simulink model "KillerWhaleModel"  (R2020b)
settings: Solver=ode15s  StartTime=0.0  StopTime=10.0  MaxStep=0.01  RelTol=1e-3
model workspace: external: MATLAB File KillerWhaleParams.m (data not in the file)
undefined symbols (not defined in the file or in its folder): frontParams, rearParams, standParams, X, Y, Z
libraries: sm_lib x4076, nesl_utility x6
(part 4 of 62)

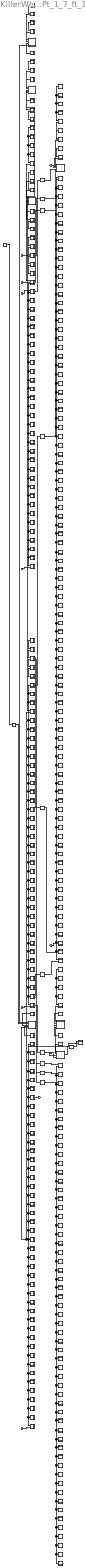
== system KillerWhaleModel/RearLinkage/Tail_Linkage_Pt_1_7_ft_1 ==
  Bracket_10_RIGID : Subsystem
  Bracket_11_RIGID : Subsystem
  Bracket_12_RIGID : Subsystem
  Bracket_13_RIGID : Subsystem
  Bracket_14_RIGID : Subsystem
  Bracket_15_RIGID : Subsystem
  Bracket_16_RIGID : Subsystem
  Bracket_17_RIGID : Subsystem
  Bracket_18_RIGID : Subsystem
  Bracket_19_RIGID : Subsystem
  Bracket_1_RIGID : Subsystem
  Bracket_1_RIGID1 : Subsystem
  Bracket_20_RIGID : Subsystem
  Bracket_21_RIGID : Subsystem
  Bracket_22_RIGID : Subsystem
  Bracket_2_RIGID : Subsystem
  Bracket_2_RIGID1 : Subsystem
  Bracket_3_RIGID : Subsystem
  Bracket_4_RIGID : Subsystem
  Bracket_5_RIGID : Subsystem
  Bracket_6_RIGID : Subsystem
  Bracket_7_RIGID : Subsystem
  Bracket_8_RIGID : Subsystem
  Bracket_9_RIGID : Subsystem
  Cylindrical3 : sm_lib/Joints/Cylindrical Joint  JointMode=Normal  SenseConstraintForce=off  SenseConstraintForceX=off  SenseConstraintForceY=off  SenseConstraintForceZ=off  SenseConstraintTorque=off  SenseConstraintTorqueX=off  SenseConstraintTorqueY=off  SenseConstraintTorqueZ=off  SenseTotalForce=off  SenseTotalForceX=off  SenseTotalForceY=off  SenseTotalForceZ=off  SenseTotalTorque=off  SenseTotalTorqueX=off  SenseTotalTorqueY=off  SenseTotalTorqueZ=off  CompositeWrenchDir=FollowerOnBase  CompositeWrenchFrame=BaseFrame  PzEquilibriumPosition=0  PzEquilibriumPositionUnits=m  PzSpringStiffness=0  PzSpringStiffnessUnits=N/m  PzDampingCoefficient=0  PzDampingCoefficientUnits=N/(m/s)  PzTorqueActuationMode=NoTorque  PzMotionActuationMode=ComputedMotion  PzSensePosition=off  PzSenseVelocity=off  PzSenseAcceleration=off  PzSenseTorqueForce=off  PzSenseLowerLimitTorqueForce=off  PzSenseUpperLimitTorqueForce=off  PzLowerLimitSpecify=off  PzLowerLimitBound=-1  PzLowerLimitBoundUnits=m  PzLowerLimitStiffness=1e6  PzLowerLimitStiffnessUnits=N/m  PzLowerLimitDamping=1e3  PzLowerLimitDampingUnits=N/(m/s)  PzLowerLimitTransitionRegionWidth=1e-4  PzLowerLimitTransitionRegionWidthUnits=m  PzUpperLimitSpecify=off  PzUpperLimitBound=1  PzUpperLimitBoundUnits=m  PzUpperLimitStiffness=1e6  PzUpperLimitStiffnessUnits=N/m  PzUpperLimitDamping=1e3  PzUpperLimitDampingUnits=N/(m/s)  PzUpperLimitTransitionRegionWidth=1e-4  PzUpperLimitTransitionRegionWidthUnits=m  PzPositionTargetSpecify=off  PzPositionTargetPriority=High  PzPositionTargetValue=0  PzPositionTargetValueUnits=m  PzVelocityTargetSpecify=off  PzVelocityTargetPriority=High  PzVelocityTargetValue=0  PzVelocityTargetValueUnits=m/s  RzEquilibriumPosition=0  RzEquilibriumPositionUnits=deg  RzSpringStiffness=0  RzSpringStiffnessUnits=N*m/deg  RzDampingCoefficient=0  RzDampingCoefficientUnits=N*m/(deg/s)  RzTorqueActuationMode=NoTorque  RzMotionActuationMode=ComputedMotion  RzSensePosition=off  RzSenseVelocity=off  RzSenseAcceleration=off  RzSenseTorqueForce=off  RzSenseLowerLimitTorqueForce=off  RzSenseUpperLimitTorqueForce=off  RzLowerLimitSpecify=off  RzLowerLimitBound=-90  RzLowerLimitBoundUnits=deg  RzLowerLimitStiffness=1e4  RzLowerLimitStiffnessUnits=N*m/deg  RzLowerLimitDamping=10  RzLowerLimitDampingUnits=N*m/(deg/s)  RzLowerLimitTransitionRegionWidth=0.1  RzLowerLimitTransitionRegionWidthUnits=deg  RzUpperLimitSpecify=off  RzUpperLimitBound=90  RzUpperLimitBoundUnits=deg  RzUpperLimitStiffness=1e4  RzUpperLimitStiffnessUnits=N*m/deg  RzUpperLimitDamping=10  RzUpperLimitDampingUnits=N*m/(deg/s)  RzUpperLimitTransitionRegionWidth=0.1  RzUpperLimitTransitionRegionWidthUnits=deg  RzPositionTargetSpecify=off  RzPositionTargetPriority=High  RzPositionTargetValue=0  RzPositionTargetValueUnits=deg  RzVelocityTargetSpecify=off  RzVelocityTargetPriority=High  RzVelocityTargetValue=0  RzVelocityTargetValueUnits=deg/s
  Cylindrical4 : sm_lib/Joints/Cylindrical Joint  JointMode=Normal  SenseConstraintForce=off  SenseConstraintForceX=off  SenseConstraintForceY=off  SenseConstraintForceZ=off  SenseConstraintTorque=off  SenseConstraintTorqueX=off  SenseConstraintTorqueY=off  SenseConstraintTorqueZ=off  SenseTotalForce=off  SenseTotalForceX=off  SenseTotalForceY=off  SenseTotalForceZ=off  SenseTotalTorque=off  SenseTotalTorqueX=off  SenseTotalTorqueY=off  SenseTotalTorqueZ=off  CompositeWrenchDir=FollowerOnBase  CompositeWrenchFrame=BaseFrame  PzEquilibriumPosition=0  PzEquilibriumPositionUnits=m  PzSpringStiffness=0  PzSpringStiffnessUnits=N/m  PzDampingCoefficient=0  PzDampingCoefficientUnits=N/(m/s)  PzTorqueActuationMode=NoTorque  PzMotionActuationMode=ComputedMotion  PzSensePosition=off  PzSenseVelocity=off  PzSenseAcceleration=off  PzSenseTorqueForce=off  PzSenseLowerLimitTorqueForce=off  PzSenseUpperLimitTorqueForce=off  PzLowerLimitSpecify=off  PzLowerLimitBound=-1  PzLowerLimitBoundUnits=m  PzLowerLimitStiffness=1e6  PzLowerLimitStiffnessUnits=N/m  PzLowerLimitDamping=1e3  PzLowerLimitDampingUnits=N/(m/s)  PzLowerLimitTransitionRegionWidth=1e-4  PzLowerLimitTransitionRegionWidthUnits=m  PzUpperLimitSpecify=off  PzUpperLimitBound=1  PzUpperLimitBoundUnits=m  PzUpperLimitStiffness=1e6  PzUpperLimitStiffnessUnits=N/m  PzUpperLimitDamping=1e3  PzUpperLimitDampingUnits=N/(m/s)  PzUpperLimitTransitionRegionWidth=1e-4  PzUpperLimitTransitionRegionWidthUnits=m  PzPositionTargetSpecify=off  PzPositionTargetPriority=High  PzPositionTargetValue=0  PzPositionTargetValueUnits=m  PzVelocityTargetSpecify=off  PzVelocityTargetPriority=High  PzVelocityTargetValue=0  PzVelocityTargetValueUnits=m/s  RzEquilibriumPosition=0  RzEquilibriumPositionUnits=deg  RzSpringStiffness=0  RzSpringStiffnessUnits=N*m/deg  RzDampingCoefficient=0  RzDampingCoefficientUnits=N*m/(deg/s)  RzTorqueActuationMode=NoTorque  RzMotionActuationMode=ComputedMotion  RzSensePosition=off  RzSenseVelocity=off  RzSenseAcceleration=off  RzSenseTorqueForce=off  RzSenseLowerLimitTorqueForce=off  RzSenseUpperLimitTorqueForce=off  RzLowerLimitSpecify=off  RzLowerLimitBound=-90  RzLowerLimitBoundUnits=deg  RzLowerLimitStiffness=1e4  RzLowerLimitStiffnessUnits=N*m/deg  RzLowerLimitDamping=10  RzLowerLimitDampingUnits=N*m/(deg/s)  RzLowerLimitTransitionRegionWidth=0.1  RzLowerLimitTransitionRegionWidthUnits=deg  RzUpperLimitSpecify=off  RzUpperLimitBound=90  RzUpperLimitBoundUnits=deg  RzUpperLimitStiffness=1e4  RzUpperLimitStiffnessUnits=N*m/deg  RzUpperLimitDamping=10  RzUpperLimitDampingUnits=N*m/(deg/s)  RzUpperLimitTransitionRegionWidth=0.1  RzUpperLimitTransitionRegionWidthUnits=deg  RzPositionTargetSpecify=off  RzPositionTargetPriority=High  RzPositionTargetValue=0  RzPositionTargetValueUnits=deg  RzVelocityTargetSpecify=off  RzVelocityTargetPriority=High  RzVelocityTargetValue=0  RzVelocityTargetValueUnits=deg/s
  Cylindrical5 : sm_lib/Joints/Cylindrical Joint  JointMode=Normal  SenseConstraintForce=off  SenseConstraintForceX=off  SenseConstraintForceY=off  SenseConstraintForceZ=off  SenseConstraintTorque=off  SenseConstraintTorqueX=off  SenseConstraintTorqueY=off  SenseConstraintTorqueZ=off  SenseTotalForce=off  SenseTotalForceX=off  SenseTotalForceY=off  SenseTotalForceZ=off  SenseTotalTorque=off  SenseTotalTorqueX=off  SenseTotalTorqueY=off  SenseTotalTorqueZ=off  CompositeWrenchDir=FollowerOnBase  CompositeWrenchFrame=BaseFrame  PzEquilibriumPosition=0  PzEquilibriumPositionUnits=m  PzSpringStiffness=0  PzSpringStiffnessUnits=N/m  PzDampingCoefficient=0  PzDampingCoefficientUnits=N/(m/s)  PzTorqueActuationMode=NoTorque  PzMotionActuationMode=ComputedMotion  PzSensePosition=off  PzSenseVelocity=off  PzSenseAcceleration=off  PzSenseTorqueForce=off  PzSenseLowerLimitTorqueForce=off  PzSenseUpperLimitTorqueForce=off  PzLowerLimitSpecify=off  PzLowerLimitBound=-1  PzLowerLimitBoundUnits=m  PzLowerLimitStiffness=1e6  PzLowerLimitStiffnessUnits=N/m  PzLowerLimitDamping=1e3  PzLowerLimitDampingUnits=N/(m/s)  PzLowerLimitTransitionRegionWidth=1e-4  PzLowerLimitTransitionRegionWidthUnits=m  PzUpperLimitSpecify=off  PzUpperLimitBound=1  PzUpperLimitBoundUnits=m  PzUpperLimitStiffness=1e6  PzUpperLimitStiffnessUnits=N/m  PzUpperLimitDamping=1e3  PzUpperLimitDampingUnits=N/(m/s)  PzUpperLimitTransitionRegionWidth=1e-4  PzUpperLimitTransitionRegionWidthUnits=m  PzPositionTargetSpecify=off  PzPositionTargetPriority=High  PzPositionTargetValue=0  PzPositionTargetValueUnits=m  PzVelocityTargetSpecify=off  PzVelocityTargetPriority=High  PzVelocityTargetValue=0  PzVelocityTargetValueUnits=m/s  RzEquilibriumPosition=0  RzEquilibriumPositionUnits=deg  RzSpringStiffness=0  RzSpringStiffnessUnits=N*m/deg  RzDampingCoefficient=0  RzDampingCoefficientUnits=N*m/(deg/s)  RzTorqueActuationMode=NoTorque  RzMotionActuationMode=ComputedMotion  RzSensePosition=off  RzSenseVelocity=off  RzSenseAcceleration=off  RzSenseTorqueForce=off  RzSenseLowerLimitTorqueForce=off  RzSenseUpperLimitTorqueForce=off  RzLowerLimitSpecify=off  RzLowerLimitBound=-90  RzLowerLimitBoundUnits=deg  RzLowerLimitStiffness=1e4  RzLowerLimitStiffnessUnits=N*m/deg  RzLowerLimitDamping=10  RzLowerLimitDampingUnits=N*m/(deg/s)  RzLowerLimitTransitionRegionWidth=0.1  RzLowerLimitTransitionRegionWidthUnits=deg  RzUpperLimitSpecify=off  RzUpperLimitBound=90  RzUpperLimitBoundUnits=deg  RzUpperLimitStiffness=1e4  RzUpperLimitStiffnessUnits=N*m/deg  RzUpperLimitDamping=10  RzUpperLimitDampingUnits=N*m/(deg/s)  RzUpperLimitTransitionRegionWidth=0.1  RzUpperLimitTransitionRegionWidthUnits=deg  RzPositionTargetSpecify=off  RzPositionTargetPriority=High  RzPositionTargetValue=0  RzPositionTargetValueUnits=deg  RzVelocityTargetSpecify=off  RzVelocityTargetPriority=High  RzVelocityTargetValue=0  RzVelocityTargetValueUnits=deg/s
  Frame_Part_1_RIGID : Subsystem
  Frame_Part_1_RIGID1 : Subsystem
  Frame_Part_1_RIGID2 : Subsystem
  Frame_Part_2_RIGID : Subsystem
  Frame_Part_2_RIGID1 : Subsystem
  Frame_Part_2_RIGID2 : Subsystem
  Hinge_10_RIGID : Subsystem
  Hinge_11_RIGID : Subsystem
  Hinge_13_RIGID : Subsystem
  Hinge_1_RIGID : Subsystem
  Hinge_1_RIGID1 : Subsystem
  Hinge_1_RIGID2 : Subsystem
  Hinge_2_RIGID : Subsystem
  Hinge_3_RIGID : Subsystem
  Hinge_4_RIGID : Subsystem
  Hinge_5_RIGID : Subsystem
  Hinge_6_RIGID : Subsystem
  Hinge_7_RIGID : Subsystem
  Hinge_8_RIGID : Subsystem
  Hinge_9_RIGID : Subsystem
  Lock_tabs_1_RIGID : Subsystem
  Lock_tabs_1_RIGID1 : Subsystem
  Lock_tabs_1_RIGID10 : Subsystem
  Lock_tabs_1_RIGID11 : Subsystem
  Lock_tabs_1_RIGID12 : Subsystem
  Lock_tabs_1_RIGID13 : Subsystem
  Lock_tabs_1_RIGID2 : Subsystem
  Lock_tabs_1_RIGID3 : Subsystem
  Lock_tabs_1_RIGID4 : Subsystem
  Lock_tabs_1_RIGID5 : Subsystem
  Lock_tabs_1_RIGID6 : Subsystem
  Lock_tabs_1_RIGID7 : Subsystem
  Lock_tabs_1_RIGID8 : Subsystem
  Lock_tabs_1_RIGID9 : Subsystem
  ReferenceFrame : sm_lib/Frames and Transforms/Reference Frame
  Revolute1 : sm_lib/Joints/Revolute Joint  JointMode=Normal  SenseConstraintForce=off  SenseConstraintForceX=off  SenseConstraintForceY=off  SenseConstraintForceZ=off  SenseConstraintTorque=off  SenseConstraintTorqueX=off  SenseConstraintTorqueY=off  SenseConstraintTorqueZ=off  SenseTotalForce=off  SenseTotalForceX=off  SenseTotalForceY=off  SenseTotalForceZ=off  SenseTotalTorque=off  SenseTotalTorqueX=off  SenseTotalTorqueY=off  SenseTotalTorqueZ=off  CompositeWrenchDir=FollowerOnBase  CompositeWrenchFrame=BaseFrame  EquilibriumPosition=0  EquilibriumPositionUnits=deg  SpringStiffness=0  SpringStiffnessUnits=N*m/deg  DampingCoefficient=0  DampingCoefficientUnits=N*m/(deg/s)  TorqueActuationMode=NoTorque  MotionActuationMode=ComputedMotion  SensePosition=off  SenseVelocity=off  SenseAcceleration=off  SenseTorqueForce=off  SenseLowerLimitTorqueForce=off  SenseUpperLimitTorqueForce=off  LowerLimitSpecify=off  LowerLimitBound=-90  LowerLimitBoundUnits=deg  LowerLimitStiffness=1e4  LowerLimitStiffnessUnits=N*m/deg  LowerLimitDamping=10  LowerLimitDampingUnits=N*m/(deg/s)  LowerLimitTransitionRegionWidth=0.1  LowerLimitTransitionRegionWidthUnits=deg  UpperLimitSpecify=off  UpperLimitBound=90  UpperLimitBoundUnits=deg  UpperLimitStiffness=1e4  UpperLimitStiffnessUnits=N*m/deg  UpperLimitDamping=10  UpperLimitDampingUnits=N*m/(deg/s)  UpperLimitTransitionRegionWidth=0.1  UpperLimitTransitionRegionWidthUnits=deg  PositionTargetSpecify=on  PositionTargetPriority=Low  PositionTargetValue=rearParams.RevoluteJoint(18).Rz.Pos  PositionTargetValueUnits=deg  VelocityTargetSpecify=off  VelocityTargetPriority=High  VelocityTargetValue=0  VelocityTargetValueUnits=deg/s
  Revolute11 : sm_lib/Joints/Revolute Joint  JointMode=Normal  SenseConstraintForce=off  SenseConstraintForceX=off  SenseConstraintForceY=off  SenseConstraintForceZ=off  SenseConstraintTorque=off  SenseConstraintTorqueX=off  SenseConstraintTorqueY=off  SenseConstraintTorqueZ=off  SenseTotalForce=off  SenseTotalForceX=off  SenseTotalForceY=off  SenseTotalForceZ=off  SenseTotalTorque=off  SenseTotalTorqueX=off  SenseTotalTorqueY=off  SenseTotalTorqueZ=off  CompositeWrenchDir=FollowerOnBase  CompositeWrenchFrame=BaseFrame  EquilibriumPosition=0  EquilibriumPositionUnits=deg  SpringStiffness=0  SpringStiffnessUnits=N*m/deg  DampingCoefficient=0  DampingCoefficientUnits=N*m/(deg/s)  TorqueActuationMode=NoTorque  MotionActuationMode=ComputedMotion  SensePosition=off  SenseVelocity=off  SenseAcceleration=off  SenseTorqueForce=off  SenseLowerLimitTorqueForce=off  SenseUpperLimitTorqueForce=off  LowerLimitSpecify=off  LowerLimitBound=-90  LowerLimitBoundUnits=deg  LowerLimitStiffness=1e4  LowerLimitStiffnessUnits=N*m/deg  LowerLimitDamping=10  LowerLimitDampingUnits=N*m/(deg/s)  LowerLimitTransitionRegionWidth=0.1  LowerLimitTransitionRegionWidthUnits=deg  UpperLimitSpecify=off  UpperLimitBound=90  UpperLimitBoundUnits=deg  UpperLimitStiffness=1e4  UpperLimitStiffnessUnits=N*m/deg  UpperLimitDamping=10  UpperLimitDampingUnits=N*m/(deg/s)  UpperLimitTransitionRegionWidth=0.1  UpperLimitTransitionRegionWidthUnits=deg  PositionTargetSpecify=on  PositionTargetPriority=Low  PositionTargetValue=rearParams.RevoluteJoint(16).Rz.Pos  PositionTargetValueUnits=deg  VelocityTargetSpecify=off  VelocityTargetPriority=High  VelocityTargetValue=0  VelocityTargetValueUnits=deg/s
  Revolute2 : sm_lib/Joints/Revolute Joint  JointMode=Normal  SenseConstraintForce=off  SenseConstraintForceX=off  SenseConstraintForceY=off  SenseConstraintForceZ=off  SenseConstraintTorque=off  SenseConstraintTorqueX=off  SenseConstraintTorqueY=off  SenseConstraintTorqueZ=off  SenseTotalForce=off  SenseTotalForceX=off  SenseTotalForceY=off  SenseTotalForceZ=off  SenseTotalTorque=off  SenseTotalTorqueX=off  SenseTotalTorqueY=off  SenseTotalTorqueZ=off  CompositeWrenchDir=FollowerOnBase  CompositeWrenchFrame=BaseFrame  EquilibriumPosition=0  EquilibriumPositionUnits=deg  SpringStiffness=0  SpringStiffnessUnits=N*m/deg  DampingCoefficient=0  DampingCoefficientUnits=N*m/(deg/s)  TorqueActuationMode=NoTorque  MotionActuationMode=ComputedMotion  SensePosition=off  SenseVelocity=off  SenseAcceleration=off  SenseTorqueForce=off  SenseLowerLimitTorqueForce=off  SenseUpperLimitTorqueForce=off  LowerLimitSpecify=off  LowerLimitBound=-90  LowerLimitBoundUnits=deg  LowerLimitStiffness=1e4  LowerLimitStiffnessUnits=N*m/deg  LowerLimitDamping=10  LowerLimitDampingUnits=N*m/(deg/s)  LowerLimitTransitionRegionWidth=0.1  LowerLimitTransitionRegionWidthUnits=deg  UpperLimitSpecify=off  UpperLimitBound=90  UpperLimitBoundUnits=deg  UpperLimitStiffness=1e4  UpperLimitStiffnessUnits=N*m/deg  UpperLimitDamping=10  UpperLimitDampingUnits=N*m/(deg/s)  UpperLimitTransitionRegionWidth=0.1  UpperLimitTransitionRegionWidthUnits=deg  PositionTargetSpecify=off  PositionTargetPriority=High  PositionTargetValue=0  PositionTargetValueUnits=deg  VelocityTargetSpecify=off  VelocityTargetPriority=High  VelocityTargetValue=0  VelocityTargetValueUnits=deg/s
  Revolute3 : sm_lib/Joints/Revolute Joint  JointMode=Normal  SenseConstraintForce=off  SenseConstraintForceX=off  SenseConstraintForceY=off  SenseConstraintForceZ=off  SenseConstraintTorque=off  SenseConstraintTorqueX=off  SenseConstraintTorqueY=off  SenseConstraintTorqueZ=off  SenseTotalForce=off  SenseTotalForceX=off  SenseTotalForceY=off  SenseTotalForceZ=off  SenseTotalTorque=off  SenseTotalTorqueX=off  SenseTotalTorqueY=off  SenseTotalTorqueZ=off  CompositeWrenchDir=FollowerOnBase  CompositeWrenchFrame=BaseFrame  EquilibriumPosition=0  EquilibriumPositionUnits=deg  SpringStiffness=0  SpringStiffnessUnits=N*m/deg  DampingCoefficient=0  DampingCoefficientUnits=N*m/(deg/s)  TorqueActuationMode=NoTorque  MotionActuationMode=ComputedMotion  SensePosition=off  SenseVelocity=off  SenseAcceleration=off  SenseTorqueForce=off  SenseLowerLimitTorqueForce=off  SenseUpperLimitTorqueForce=off  LowerLimitSpecify=off  LowerLimitBound=-90  LowerLimitBoundUnits=deg  LowerLimitStiffness=1e4  LowerLimitStiffnessUnits=N*m/deg  LowerLimitDamping=10  LowerLimitDampingUnits=N*m/(deg/s)  LowerLimitTransitionRegionWidth=0.1  LowerLimitTransitionRegionWidthUnits=deg  UpperLimitSpecify=off  UpperLimitBound=90  UpperLimitBoundUnits=deg  UpperLimitStiffness=1e4  UpperLimitStiffnessUnits=N*m/deg  UpperLimitDamping=10  UpperLimitDampingUnits=N*m/(deg/s)  UpperLimitTransitionRegionWidth=0.1  UpperLimitTransitionRegionWidthUnits=deg  PositionTargetSpecify=on  PositionTargetPriority=Low  PositionTargetValue=rearParams.RevoluteJoint(15).Rz.Pos  PositionTargetValueUnits=deg  VelocityTargetSpecify=off  VelocityTargetPriority=High  VelocityTargetValue=0  VelocityTargetValueUnits=deg/s
  Revolute4 : sm_lib/Joints/Revolute Joint  JointMode=Normal  SenseConstraintForce=off  SenseConstraintForceX=off  SenseConstraintForceY=off  SenseConstraintForceZ=off  SenseConstraintTorque=off  SenseConstraintTorqueX=off  SenseConstraintTorqueY=off  SenseConstraintTorqueZ=off  SenseTotalForce=off  SenseTotalForceX=off  SenseTotalForceY=off  SenseTotalForceZ=off  SenseTotalTorque=off  SenseTotalTorqueX=off  SenseTotalTorqueY=off  SenseTotalTorqueZ=off  CompositeWrenchDir=FollowerOnBase  CompositeWrenchFrame=BaseFrame  EquilibriumPosition=0  EquilibriumPositionUnits=deg  SpringStiffness=0  SpringStiffnessUnits=N*m/deg  DampingCoefficient=0  DampingCoefficientUnits=N*m/(deg/s)  TorqueActuationMode=NoTorque  MotionActuationMode=ComputedMotion  SensePosition=off  SenseVelocity=off  SenseAcceleration=off  SenseTorqueForce=off  SenseLowerLimitTorqueForce=off  SenseUpperLimitTorqueForce=off  LowerLimitSpecify=off  LowerLimitBound=-90  LowerLimitBoundUnits=deg  LowerLimitStiffness=1e4  LowerLimitStiffnessUnits=N*m/deg  LowerLimitDamping=10  LowerLimitDampingUnits=N*m/(deg/s)  LowerLimitTransitionRegionWidth=0.1  LowerLimitTransitionRegionWidthUnits=deg  UpperLimitSpecify=off  UpperLimitBound=90  UpperLimitBoundUnits=deg  UpperLimitStiffness=1e4  UpperLimitStiffnessUnits=N*m/deg  UpperLimitDamping=10  UpperLimitDampingUnits=N*m/(deg/s)  UpperLimitTransitionRegionWidth=0.1  UpperLimitTransitionRegionWidthUnits=deg  PositionTargetSpecify=on  PositionTargetPriority=Low  PositionTargetValue=rearParams.RevoluteJoint(20).Rz.Pos  PositionTargetValueUnits=deg  VelocityTargetSpecify=off  VelocityTargetPriority=High  VelocityTargetValue=0  VelocityTargetValueUnits=deg/s
  Revolute5 : sm_lib/Joints/Revolute Joint  JointMode=Normal  SenseConstraintForce=off  SenseConstraintForceX=off  SenseConstraintForceY=off  SenseConstraintForceZ=off  SenseConstraintTorque=off  SenseConstraintTorqueX=off  SenseConstraintTorqueY=off  SenseConstraintTorqueZ=off  SenseTotalForce=off  SenseTotalForceX=off  SenseTotalForceY=off  SenseTotalForceZ=off  SenseTotalTorque=off  SenseTotalTorqueX=off  SenseTotalTorqueY=off  SenseTotalTorqueZ=off  CompositeWrenchDir=FollowerOnBase  CompositeWrenchFrame=BaseFrame  EquilibriumPosition=0  EquilibriumPositionUnits=deg  SpringStiffness=0  SpringStiffnessUnits=N*m/deg  DampingCoefficient=0  DampingCoefficientUnits=N*m/(deg/s)  TorqueActuationMode=NoTorque  MotionActuationMode=ComputedMotion  SensePosition=off  SenseVelocity=off  SenseAcceleration=off  SenseTorqueForce=off  SenseLowerLimitTorqueForce=off  SenseUpperLimitTorqueForce=off  LowerLimitSpecify=off  LowerLimitBound=-90  LowerLimitBoundUnits=deg  LowerLimitStiffness=1e4  LowerLimitStiffnessUnits=N*m/deg  LowerLimitDamping=10  LowerLimitDampingUnits=N*m/(deg/s)  LowerLimitTransitionRegionWidth=0.1  LowerLimitTransitionRegionWidthUnits=deg  UpperLimitSpecify=off  UpperLimitBound=90  UpperLimitBoundUnits=deg  UpperLimitStiffness=1e4  UpperLimitStiffnessUnits=N*m/deg  UpperLimitDamping=10  UpperLimitDampingUnits=N*m/(deg/s)  UpperLimitTransitionRegionWidth=0.1  UpperLimitTransitionRegionWidthUnits=deg  PositionTargetSpecify=on  PositionTargetPriority=Low  PositionTargetValue=rearParams.RevoluteJoint(14).Rz.Pos  PositionTargetValueUnits=deg  VelocityTargetSpecify=off  VelocityTargetPriority=High  VelocityTargetValue=0  VelocityTargetValueUnits=deg/s
  Revolute6 : sm_lib/Joints/Revolute Joint  JointMode=Normal  SenseConstraintForce=off  SenseConstraintForceX=off  SenseConstraintForceY=off  SenseConstraintForceZ=off  SenseConstraintTorque=off  SenseConstraintTorqueX=off  SenseConstraintTorqueY=off  SenseConstraintTorqueZ=off  SenseTotalForce=off  SenseTotalForceX=off  SenseTotalForceY=off  SenseTotalForceZ=off  SenseTotalTorque=off  SenseTotalTorqueX=off  SenseTotalTorqueY=off  SenseTotalTorqueZ=off  CompositeWrenchDir=FollowerOnBase  CompositeWrenchFrame=BaseFrame  EquilibriumPosition=0  EquilibriumPositionUnits=deg  SpringStiffness=0  SpringStiffnessUnits=N*m/deg  DampingCoefficient=0  DampingCoefficientUnits=N*m/(deg/s)  TorqueActuationMode=NoTorque  MotionActuationMode=ComputedMotion  SensePosition=off  SenseVelocity=off  SenseAcceleration=off  SenseTorqueForce=off  SenseLowerLimitTorqueForce=off  SenseUpperLimitTorqueForce=off  LowerLimitSpecify=off  LowerLimitBound=-90  LowerLimitBoundUnits=deg  LowerLimitStiffness=1e4  LowerLimitStiffnessUnits=N*m/deg  LowerLimitDamping=10  LowerLimitDampingUnits=N*m/(deg/s)  LowerLimitTransitionRegionWidth=0.1  LowerLimitTransitionRegionWidthUnits=deg  UpperLimitSpecify=off  UpperLimitBound=90  UpperLimitBoundUnits=deg  UpperLimitStiffness=1e4  UpperLimitStiffnessUnits=N*m/deg  UpperLimitDamping=10  UpperLimitDampingUnits=N*m/(deg/s)  UpperLimitTransitionRegionWidth=0.1  UpperLimitTransitionRegionWidthUnits=deg  PositionTargetSpecify=on  PositionTargetPriority=Low  PositionTargetValue=rearParams.RevoluteJoint(21).Rz.Pos  PositionTargetValueUnits=deg  VelocityTargetSpecify=off  VelocityTargetPriority=High  VelocityTargetValue=0  VelocityTargetValueUnits=deg/s
  Revolute7 : sm_lib/Joints/Revolute Joint  JointMode=Normal  SenseConstraintForce=off  SenseConstraintForceX=off  SenseConstraintForceY=off  SenseConstraintForceZ=off  SenseConstraintTorque=off  SenseConstraintTorqueX=off  SenseConstraintTorqueY=off  SenseConstraintTorqueZ=off  SenseTotalForce=off  SenseTotalForceX=off  SenseTotalForceY=off  SenseTotalForceZ=off  SenseTotalTorque=off  SenseTotalTorqueX=off  SenseTotalTorqueY=off  SenseTotalTorqueZ=off  CompositeWrenchDir=FollowerOnBase  CompositeWrenchFrame=BaseFrame  EquilibriumPosition=0  EquilibriumPositionUnits=deg  SpringStiffness=0  SpringStiffnessUnits=N*m/deg  DampingCoefficient=0  DampingCoefficientUnits=N*m/(deg/s)  TorqueActuationMode=NoTorque  MotionActuationMode=ComputedMotion  SensePosition=off  SenseVelocity=off  SenseAcceleration=off  SenseTorqueForce=off  SenseLowerLimitTorqueForce=off  SenseUpperLimitTorqueForce=off  LowerLimitSpecify=off  LowerLimitBound=-90  LowerLimitBoundUnits=deg  LowerLimitStiffness=1e4  LowerLimitStiffnessUnits=N*m/deg  LowerLimitDamping=10  LowerLimitDampingUnits=N*m/(deg/s)  LowerLimitTransitionRegionWidth=0.1  LowerLimitTransitionRegionWidthUnits=deg  UpperLimitSpecify=off  UpperLimitBound=90  UpperLimitBoundUnits=deg  UpperLimitStiffness=1e4  UpperLimitStiffnessUnits=N*m/deg  UpperLimitDamping=10  UpperLimitDampingUnits=N*m/(deg/s)  UpperLimitTransitionRegionWidth=0.1  UpperLimitTransitionRegionWidthUnits=deg  PositionTargetSpecify=on  PositionTargetPriority=Low  PositionTargetValue=rearParams.RevoluteJoint(19).Rz.Pos  PositionTargetValueUnits=deg  VelocityTargetSpecify=off  VelocityTargetPriority=High  VelocityTargetValue=0  VelocityTargetValueUnits=deg/s
  Screw_10_3_4_in_1_RIGID : Subsystem
  Screw_10_3_4_in_1_RIGID1 : Subsystem
  Screw_10_3_4_in_1_RIGID2 : Subsystem
  Screw_10_3_4_in_1_RIGID3 : Subsystem
  Screw_8_1_2_in_1_RIGID : Subsystem
  Screw_8_1_2_in_1_RIGID1 : Subsystem
  Screw_8_1_2_in_1_RIGID10 : Subsystem
  Screw_8_1_2_in_1_RIGID11 : Subsystem
  Screw_8_1_2_in_1_RIGID12 : Subsystem
  Screw_8_1_2_in_1_RIGID13 : Subsystem
  Screw_8_1_2_in_1_RIGID14 : Subsystem
  Screw_8_1_2_in_1_RIGID15 : Subsystem
  Screw_8_1_2_in_1_RIGID16 : Subsystem
  Screw_8_1_2_in_1_RIGID17 : Subsystem
  Screw_8_1_2_in_1_RIGID18 : Subsystem
  Screw_8_1_2_in_1_RIGID19 : Subsystem
  Screw_8_1_2_in_1_RIGID2 : Subsystem
  Screw_8_1_2_in_1_RIGID3 : Subsystem
  Screw_8_1_2_in_1_RIGID4 : Subsystem
  Screw_8_1_2_in_1_RIGID5 : Subsystem
  Screw_8_1_2_in_1_RIGID6 : Subsystem
  Screw_8_1_2_in_1_RIGID7 : Subsystem
  Screw_8_1_2_in_1_RIGID8 : Subsystem
  Screw_8_1_2_in_1_RIGID9 : Subsystem
  Screw_8_3_4_in_1_RIGID : Subsystem
  Screw_8_3_4_in_1_RIGID1 : Subsystem
  Screw_8_3_4_in_1_RIGID2 : Subsystem
  Screw_8_3_4_in_1_RIGID3 : Subsystem
  Screw_8_3_4_in_1_RIGID4 : Subsystem
  Screw_8_3_4_in_1_RIGID5 : Subsystem
  Set_Screw_4_1_4_in_10_RIGID : Subsystem
  Set_Screw_4_1_4_in_11_RIGID : Subsystem
  Set_Screw_4_1_4_in_12_RIGID : Subsystem
  Set_Screw_4_1_4_in_13_RIGID : Subsystem
  Set_Screw_4_1_4_in_14_RIGID : Subsystem
  Set_Screw_4_1_4_in_15_RIGID : Subsystem
  Set_Screw_4_1_4_in_16_RIGID : Subsystem
  Set_Screw_4_1_4_in_17_RIGID : Subsystem
  Set_Screw_4_1_4_in_18_RIGID : Subsystem
  Set_Screw_4_1_4_in_19_RIGID : Subsystem
  Set_Screw_4_1_4_in_1_RIGID : Subsystem
  Set_Screw_4_1_4_in_20_RIGID : Subsystem
  Set_Screw_4_1_4_in_21_RIGID : Subsystem
  Set_Screw_4_1_4_in_22_RIGID : Subsystem
  Set_Screw_4_1_4_in_23_RIGID : Subsystem
  Set_Screw_4_1_4_in_24_RIGID : Subsystem
  Set_Screw_4_1_4_in_2_RIGID : Subsystem
  Set_Screw_4_1_4_in_3_RIGID : Subsystem
  Set_Screw_4_1_4_in_4_RIGID : Subsystem
  Set_Screw_4_1_4_in_5_RIGID : Subsystem
  Set_Screw_4_1_4_in_6_RIGID : Subsystem
  Set_Screw_4_1_4_in_7_RIGID : Subsystem
  Set_Screw_4_1_4_in_8_RIGID : Subsystem
  Set_Screw_4_1_4_in_9_RIGID : Subsystem
  Spacer_1_RIGID : Subsystem
  Spacer_1_RIGID1 : Subsystem
  Spacer_1_RIGID10 : Subsystem
  Spacer_1_RIGID11 : Subsystem
  Spacer_1_RIGID12 : Subsystem
  Spacer_1_RIGID13 : Subsystem
  Spacer_1_RIGID14 : Subsystem
  Spacer_1_RIGID15 : Subsystem
  Spacer_1_RIGID16 : Subsystem
  Spacer_1_RIGID17 : Subsystem
  Spacer_1_RIGID18 : Subsystem
  Spacer_1_RIGID19 : Subsystem
  Spacer_1_RIGID2 : Subsystem
  Spacer_1_RIGID20 : Subsystem
  Spacer_1_RIGID21 : Subsystem
  Spacer_1_RIGID22 : Subsystem
  Spacer_1_RIGID23 : Subsystem
  Spacer_1_RIGID24 : Subsystem
  Spacer_1_RIGID25 : Subsystem
  Spacer_1_RIGID3 : Subsystem
  Spacer_1_RIGID4 : Subsystem
  Spacer_1_RIGID5 : Subsystem
  Spacer_1_RIGID6 : Subsystem
  Spacer_1_RIGID7 : Subsystem
  Spacer_1_RIGID8 : Subsystem
  Spacer_1_RIGID9 : Subsystem
  Spacer_2_RIGID : Subsystem
  Spacer_3_RIGID : Subsystem
  Spring_Pin_1_8_in_OD_1_4_in_L_10_RIGID : Subsystem
  Spring_Pin_1_8_in_OD_1_4_in_L_10_RIGID1 : Subsystem
  Spring_Pin_1_8_in_OD_1_4_in_L_10_RIGID2 : Subsystem
  Spring_Pin_1_8_in_OD_1_4_in_L_10_RIGID3 : Subsystem
  Spring_Pin_1_8_in_OD_1_4_in_L_11_RIGID : Subsystem
  Spring_Pin_1_8_in_OD_1_4_in_L_11_RIGID1 : Subsystem
  Spring_Pin_1_8_in_OD_1_4_in_L_11_RIGID2 : Subsystem
  Spring_Pin_1_8_in_OD_1_4_in_L_11_RIGID3 : Subsystem
  Spring_Pin_1_8_in_OD_1_4_in_L_12_RIGID : Subsystem
  Spring_Pin_1_8_in_OD_1_4_in_L_12_RIGID1 : Subsystem
  Spring_Pin_1_8_in_OD_1_4_in_L_12_RIGID2 : Subsystem
  Spring_Pin_1_8_in_OD_1_4_in_L_12_RIGID3 : Subsystem
  Spring_Pin_1_8_in_OD_1_4_in_L_13_RIGID : Subsystem
  Spring_Pin_1_8_in_OD_1_4_in_L_13_RIGID1 : Subsystem
  Spring_Pin_1_8_in_OD_1_4_in_L_13_RIGID2 : Subsystem
  Spring_Pin_1_8_in_OD_1_4_in_L_14_RIGID : Subsystem
  Spring_Pin_1_8_in_OD_1_4_in_L_14_RIGID1 : Subsystem
  Spring_Pin_1_8_in_OD_1_4_in_L_14_RIGID2 : Subsystem
  Spring_Pin_1_8_in_OD_1_4_in_L_15_RIGID : Subsystem
  Spring_Pin_1_8_in_OD_1_4_in_L_15_RIGID1 : Subsystem
  Spring_Pin_1_8_in_OD_1_4_in_L_15_RIGID2 : Subsystem
  Spring_Pin_1_8_in_OD_1_4_in_L_16_RIGID : Subsystem
  Spring_Pin_1_8_in_OD_1_4_in_L_16_RIGID1 : Subsystem
  Spring_Pin_1_8_in_OD_1_4_in_L_16_RIGID2 : Subsystem
  Spring_Pin_1_8_in_OD_1_4_in_L_17_RIGID : Subsystem
  Spring_Pin_1_8_in_OD_1_4_in_L_17_RIGID1 : Subsystem
  Spring_Pin_1_8_in_OD_1_4_in_L_17_RIGID2 : Subsystem
  Spring_Pin_1_8_in_OD_1_4_in_L_18_RIGID : Subsystem
  Spring_Pin_1_8_in_OD_1_4_in_L_18_RIGID1 : Subsystem
  Spring_Pin_1_8_in_OD_1_4_in_L_18_RIGID2 : Subsystem
  Spring_Pin_1_8_in_OD_1_4_in_L_19_RIGID : Subsystem
  Spring_Pin_1_8_in_OD_1_4_in_L_19_RIGID1 : Subsystem
  Spring_Pin_1_8_in_OD_1_4_in_L_19_RIGID2 : Subsystem
  Spring_Pin_1_8_in_OD_1_4_in_L_1_RIGID : Subsystem
  Spring_Pin_1_8_in_OD_1_4_in_L_1_RIGID1 : Subsystem
  Spring_Pin_1_8_in_OD_1_4_in_L_1_RIGID2 : Subsystem
  Spring_Pin_1_8_in_OD_1_4_in_L_20_RIGID : Subsystem
  Spring_Pin_1_8_in_OD_1_4_in_L_20_RIGID1 : Subsystem
  Spring_Pin_1_8_in_OD_1_4_in_L_20_RIGID2 : Subsystem
  Spring_Pin_1_8_in_OD_1_4_in_L_21_RIGID : Subsystem
  Spring_Pin_1_8_in_OD_1_4_in_L_22_RIGID : Subsystem
  Spring_Pin_1_8_in_OD_1_4_in_L_2_RIGID : Subsystem
  Spring_Pin_1_8_in_OD_1_4_in_L_2_RIGID1 : Subsystem
  Spring_Pin_1_8_in_OD_1_4_in_L_2_RIGID2 : Subsystem
  Spring_Pin_1_8_in_OD_1_4_in_L_3_RIGID : Subsystem
  Spring_Pin_1_8_in_OD_1_4_in_L_3_RIGID1 : Subsystem
  Spring_Pin_1_8_in_OD_1_4_in_L_3_RIGID2 : Subsystem
  Spring_Pin_1_8_in_OD_1_4_in_L_3_RIGID3 : Subsystem
  Spring_Pin_1_8_in_OD_1_4_in_L_4_RIGID : Subsystem
  Spring_Pin_1_8_in_OD_1_4_in_L_4_RIGID1 : Subsystem
  Spring_Pin_1_8_in_OD_1_4_in_L_4_RIGID2 : Subsystem
  Spring_Pin_1_8_in_OD_1_4_in_L_4_RIGID3 : Subsystem
  Spring_Pin_1_8_in_OD_1_4_in_L_5_RIGID : Subsystem
  Spring_Pin_1_8_in_OD_1_4_in_L_5_RIGID1 : Subsystem
  Spring_Pin_1_8_in_OD_1_4_in_L_5_RIGID2 : Subsystem
  Spring_Pin_1_8_in_OD_1_4_in_L_5_RIGID3 : Subsystem
  Spring_Pin_1_8_in_OD_1_4_in_L_6_RIGID : Subsystem
  Spring_Pin_1_8_in_OD_1_4_in_L_6_RIGID1 : Subsystem
  Spring_Pin_1_8_in_OD_1_4_in_L_6_RIGID2 : Subsystem
  Spring_Pin_1_8_in_OD_1_4_in_L_6_RIGID3 : Subsystem
  Spring_Pin_1_8_in_OD_1_4_in_L_7_RIGID : Subsystem
  Spring_Pin_1_8_in_OD_1_4_in_L_7_RIGID1 : Subsystem
  Spring_Pin_1_8_in_OD_1_4_in_L_7_RIGID2 : Subsystem
  Spring_Pin_1_8_in_OD_1_4_in_L_7_RIGID3 : Subsystem
  Spring_Pin_1_8_in_OD_1_4_in_L_8_RIGID : Subsystem
  Spring_Pin_1_8_in_OD_1_4_in_L_8_RIGID1 : Subsystem
  Spring_Pin_1_8_in_OD_1_4_in_L_8_RIGID2 : Subsystem
  Spring_Pin_1_8_in_OD_1_4_in_L_8_RIGID3 : Subsystem
  Spring_Pin_1_8_in_OD_1_4_in_L_9_RIGID : Subsystem
  Spring_Pin_1_8_in_OD_1_4_in_L_9_RIGID1 : Subsystem
  Spring_Pin_1_8_in_OD_1_4_in_L_9_RIGID2 : Subsystem
  Spring_Pin_1_8_in_OD_1_4_in_L_9_RIGID3 : Subsystem
  Spring_Pin_3_32_in_OD_3_16_in_L_1_RIGID : Subsystem
  Spring_Pin_3_32_in_OD_3_16_in_L_1_RIGID1 : Subsystem
  Spring_Pin_3_32_in_OD_3_16_in_L_1_RIGID10 : Subsystem
  Spring_Pin_3_32_in_OD_3_16_in_L_1_RIGID11 : Subsystem
  Spring_Pin_3_32_in_OD_3_16_in_L_1_RIGID2 : Subsystem
  Spring_Pin_3_32_in_OD_3_16_in_L_1_RIGID3 : Subsystem
  Spring_Pin_3_32_in_OD_3_16_in_L_1_RIGID4 : Subsystem
  Spring_Pin_3_32_in_OD_3_16_in_L_1_RIGID5 : Subsystem
  Spring_Pin_3_32_in_OD_3_16_in_L_1_RIGID6 : Subsystem
  Spring_Pin_3_32_in_OD_3_16_in_L_1_RIGID7 : Subsystem
  Spring_Pin_3_32_in_OD_3_16_in_L_1_RIGID8 : Subsystem
  Spring_Pin_3_32_in_OD_3_16_in_L_1_RIGID9 : Subsystem
  Standoff_1_RIGID : Subsystem
  Standoff_1_RIGID1 : Subsystem
  Standoff_2_RIGID : Subsystem
  Standoff_3_RIGID : Subsystem
  Transform : sm_lib/Frames and Transforms/Rigid Transform  TranslationMethod=Cartesian  TranslationStandardOffset=0  TranslationLengthUnit=in  TranslationStandardAxis=+Z  TranslationCartesianOffset=rearParams.RigidTransform(790).translation  TranslationROffset=0  TranslationROffsetUnits=m  TranslationZOffset=0  TranslationZOffsetUnits=m  TranslationThetaOffset=0  TranslationThetaOffsetUnits=deg  RotationMethod=ArbitraryAxis  RotationAngleUnits=rad  RotationStandardAxis=+Z  RotationAngle=rearParams.RigidTransform(790).angle  RotationArbitraryAxis=rearParams.RigidTransform(790).axis  FollAlignAxisA=+X  BaseAlignAxisA=+Y  FollAlignAxisB=+Y  BaseAlignAxisB=+Z  RotationSequenceAxes=FollowerAxes  RotationSequence=XYX  RotationSequenceAngles=[0 0 0]  RotationSequenceAnglesUnits=deg  RotationMatrix=[1 0 0; 0 1 0; 0 0 1]
  Washer_10_1_RIGID : Subsystem
  Washer_10_3_RIGID : Subsystem
  Washer_10_4_RIGID : Subsystem
  Washer_10_6_RIGID : Subsystem
  Washer_8_1_RIGID : Subsystem
  Washer_8_1_RIGID1 : Subsystem
  Washer_8_1_RIGID10 : Subsystem
  Washer_8_1_RIGID11 : Subsystem
  Washer_8_1_RIGID12 : Subsystem
  Washer_8_1_RIGID13 : Subsystem
  Washer_8_1_RIGID14 : Subsystem
  Washer_8_1_RIGID15 : Subsystem
  Washer_8_1_RIGID16 : Subsystem
  Washer_8_1_RIGID17 : Subsystem
  Washer_8_1_RIGID18 : Subsystem
  Washer_8_1_RIGID19 : Subsystem
  Washer_8_1_RIGID2 : Subsystem
  Washer_8_1_RIGID20 : Subsystem
  Washer_8_1_RIGID21 : Subsystem
  Washer_8_1_RIGID22 : Subsystem
  Washer_8_1_RIGID23 : Subsystem
  Washer_8_1_RIGID24 : Subsystem
  Washer_8_1_RIGID25 : Subsystem
  Washer_8_1_RIGID3 : Subsystem
  Washer_8_1_RIGID4 : Subsystem
  Washer_8_1_RIGID5 : Subsystem
  Washer_8_1_RIGID6 : Subsystem
  Washer_8_1_RIGID7 : Subsystem
  Washer_8_1_RIGID8 : Subsystem
  Washer_8_1_RIGID9 : Subsystem
  bracesb1_1_RIGID : Subsystem
  bracesb1_2_RIGID : Subsystem
  bracesb1_3_RIGID : Subsystem
  bracesb1_4_RIGID : Subsystem
  bracesb1_5_RIGID : Subsystem
  bracesb1_6_RIGID : Subsystem
  bracesb1_7_RIGID : Subsystem
  bracesb2_1_RIGID : Subsystem
  bracesb2_2_RIGID : Subsystem
  bracesb2_3_RIGID : Subsystem
  bracesb3_1_RIGID : Subsystem
  bracesb3_2_RIGID : Subsystem
  bracesb3_3_RIGID : Subsystem
  bracesb4_1_RIGID : Subsystem
  bracesb4_2_RIGID : Subsystem
  bracesb4_3_RIGID : Subsystem
  bracesb5_1_RIGID : Subsystem
  bracesb5_2_RIGID : Subsystem
  bracesb5_3_RIGID : Subsystem
  bracesb6_1_RIGID : Subsystem
  bracesb6_2_RIGID : Subsystem
  bracesb6_4_RIGID : Subsystem
  bracesb6_5_RIGID : Subsystem
  bracesb6_6_RIGID : Subsystem
  bracesb6_7_RIGID : Subsystem
  bracesb6_8_RIGID : Subsystem
  bracesb7_1_RIGID : Subsystem
  bracesb7_2_RIGID : Subsystem
  bracesb7_3_RIGID : Subsystem
  bracesb7_4_RIGID : Subsystem
  bracesb7_5_RIGID : Subsystem
  bracesb7_6_RIGID : Subsystem
  bracesb7_7_RIGID : Subsystem
  bracesb7_8_RIGID : Subsystem
  bulkheads2_1_RIGID : Subsystem
  bulkheads2_2_RIGID : Subsystem
  bulkheads2_3_RIGID : Subsystem
  bulkheads2_4_RIGID : Subsystem
  bulkheads2_5_RIGID : Subsystem
  bulkheads3_1_RIGID : Subsystem
  bulkheads3_2_RIGID : Subsystem
  bulkheads3_3_RIGID : Subsystem
  bulkheads3_4_RIGID : Subsystem
  bulkheads3_5_RIGID : Subsystem
  bulkheads4_1_RIGID : Subsystem
  bulkheads4_2_RIGID : Subsystem
  bulkheads4_3_RIGID : Subsystem
  bulkheads4_4_RIGID : Subsystem
  bulkheads4_5_RIGID : Subsystem
  link1l_1_RIGID : Subsystem
  link1r_1_RIGID : Subsystem
  link2l_1_RIGID : Subsystem
  link2r_1_RIGID : Subsystem
  link3l_1_RIGID : Subsystem
  link3r_1_RIGID : Subsystem
  link4l_1_RIGID : Subsystem
  link4r_1_RIGID : Subsystem
  link5l_1_RIGID : Subsystem
  link5r_1_RIGID : Subsystem
  rear_torso_l_1_RIGID : Subsystem
  rear_torso_r_1_RIGID : Subsystem
  F4 : PMIOPort  Side=Left
  F6 : PMIOPort  Port=2  Side=Left
  F3 : PMIOPort  Port=3  Side=Left
  F2 : PMIOPort  Port=4  Side=Left
  F : PMIOPort  Port=5  Side=Left
  F8 : PMIOPort  Port=6  Side=Right
  F7 : PMIOPort  Port=7  Side=Right
  F5 : PMIOPort  Port=8  Side=Right
  F1 : PMIOPort  Port=9  Side=Right
  S4 : PMIOPort  Port=10  Side=Right
  connections:
  link3l_1_RIGID/LConn2 -- link3r_1_RIGID/LConn2
  bulkheads3_2_RIGID/LConn1 -- bulkheads3_1_RIGID/LConn1 -- bulkheads3_5_RIGID/LConn1 -- bulkheads3_4_RIGID/LConn1 -- bulkheads3_3_RIGID/LConn1
  Bracket_2_RIGID1/LConn1 -- Spacer_3_RIGID/LConn1 -- Spring_Pin_1_8_in_OD_1_4_in_L_11_RIGID/LConn1 -- Spacer_2_RIGID/LConn1 -- Spacer_1_RIGID6/LConn1 -- Spacer_1_RIGID23/LConn1 -- Spacer_1_RIGID2/LConn1 -- Spacer_1_RIGID18/LConn1 -- Spacer_1_RIGID1/LConn1 -- Set_Screw_4_1_4_in_8_RIGID/LConn1 -- Set_Screw_4_1_4_in_5_RIGID/LConn1 -- Set_Screw_4_1_4_in_4_RIGID/LConn1 -- Set_Screw_4_1_4_in_15_RIGID/LConn1 -- Screw_8_1_2_in_1_RIGID4/LConn1 -- Screw_8_1_2_in_1_RIGID/LConn1 -- Screw_10_3_4_in_1_RIGID3/LConn1 -- Screw_10_3_4_in_1_RIGID2/LConn1 -- Screw_10_3_4_in_1_RIGID1/LConn1 -- Screw_10_3_4_in_1_RIGID/LConn1 -- Hinge_2_RIGID/LConn1 -- Bracket_7_RIGID/LConn1 -- Bracket_5_RIGID/LConn1 -- Hinge_3_RIGID/LConn1 -- Spring_Pin_1_8_in_OD_1_4_in_L_11_RIGID1/LConn1 -- Spring_Pin_1_8_in_OD_1_4_in_L_1_RIGID/LConn1 -- Spring_Pin_1_8_in_OD_1_4_in_L_1_RIGID1/LConn1 -- Spring_Pin_1_8_in_OD_1_4_in_L_2_RIGID1/LConn1 -- Spring_Pin_1_8_in_OD_1_4_in_L_3_RIGID1/LConn1 -- Spring_Pin_1_8_in_OD_1_4_in_L_3_RIGID2/LConn1 -- Spring_Pin_1_8_in_OD_1_4_in_L_4_RIGID2/LConn1 -- Spring_Pin_1_8_in_OD_1_4_in_L_6_RIGID/LConn1 -- Spring_Pin_1_8_in_OD_1_4_in_L_7_RIGID1/LConn1 -- Spring_Pin_1_8_in_OD_1_4_in_L_7_RIGID2/LConn1 -- Spring_Pin_1_8_in_OD_1_4_in_L_8_RIGID2/LConn1 -- Standoff_1_RIGID1/LConn1 -- Standoff_2_RIGID/LConn1 -- Standoff_3_RIGID/LConn1 -- Washer_10_1_RIGID/LConn1 -- Washer_10_3_RIGID/LConn1 -- Washer_10_4_RIGID/LConn1 -- Washer_10_6_RIGID/LConn1 -- Washer_8_1_RIGID17/LConn1 -- Washer_8_1_RIGID9/LConn1 -- rear_torso_l_1_RIGID/LConn5 -- rear_torso_r_1_RIGID/LConn2 -- Bracket_1_RIGID1/LConn1 -- Spacer_1_RIGID9/LConn2
  link1l_1_RIGID/LConn2 -- link1r_1_RIGID/LConn1
  bracesb6_1_RIGID/LConn3 -- bracesb6_2_RIGID/LConn1
  bracesb3_3_RIGID/LConn1 -- link3r_1_RIGID/LConn1
  bracesb7_1_RIGID/LConn4 -- bracesb7_3_RIGID/LConn1
  bracesb7_1_RIGID/LConn5 -- rear_torso_r_1_RIGID/LConn1
  bracesb7_1_RIGID/LConn1 -- bracesb7_5_RIGID/LConn2
  bracesb7_1_RIGID/LConn3 -- bracesb7_8_RIGID/LConn1
  bracesb7_1_RIGID/LConn2 -- bracesb7_2_RIGID/LConn1
  Revolute5/LConn1 -- Spacer_1_RIGID3/RConn1
  Bracket_2_RIGID/LConn1 -- Bracket_12_RIGID/LConn1 -- Frame_Part_2_RIGID1/LConn1 -- Spacer_1_RIGID12/LConn1 -- Bracket_3_RIGID/LConn1 -- Bracket_9_RIGID/LConn1 -- Frame_Part_1_RIGID/LConn1 -- Washer_8_1_RIGID7/LConn1 -- Hinge_5_RIGID/LConn1 -- Hinge_7_RIGID/LConn1 -- Screw_8_1_2_in_1_RIGID1/LConn1 -- Screw_8_1_2_in_1_RIGID14/LConn1 -- Screw_8_1_2_in_1_RIGID19/LConn1 -- Screw_8_1_2_in_1_RIGID3/LConn1 -- Set_Screw_4_1_4_in_17_RIGID/LConn1 -- Set_Screw_4_1_4_in_1_RIGID/LConn1 -- Set_Screw_4_1_4_in_20_RIGID/LConn1 -- Set_Screw_4_1_4_in_9_RIGID/LConn1 -- Spacer_1_RIGID11/LConn1 -- Spacer_1_RIGID7/LConn1 -- Spring_Pin_1_8_in_OD_1_4_in_L_11_RIGID3/LConn1 -- Spring_Pin_1_8_in_OD_1_4_in_L_12_RIGID1/LConn1 -- Spring_Pin_1_8_in_OD_1_4_in_L_12_RIGID2/LConn1 -- Spring_Pin_1_8_in_OD_1_4_in_L_13_RIGID1/LConn1 -- Spring_Pin_1_8_in_OD_1_4_in_L_16_RIGID2/LConn1 -- Spring_Pin_1_8_in_OD_1_4_in_L_17_RIGID/LConn1 -- Spring_Pin_1_8_in_OD_1_4_in_L_17_RIGID1/LConn1 -- Spring_Pin_1_8_in_OD_1_4_in_L_18_RIGID1/LConn1 -- Spring_Pin_1_8_in_OD_1_4_in_L_19_RIGID/LConn1 -- Spring_Pin_1_8_in_OD_1_4_in_L_4_RIGID1/LConn1 -- Spring_Pin_1_8_in_OD_1_4_in_L_8_RIGID3/LConn1 -- Spring_Pin_1_8_in_OD_1_4_in_L_9_RIGID3/LConn1 -- Washer_8_1_RIGID11/LConn1 -- Washer_8_1_RIGID20/LConn1 -- Washer_8_1_RIGID4/LConn1 -- Spacer_1_RIGID25/LConn1
  Revolute5/RConn1 -- link3l_1_RIGID/LConn4
  bracesb1_1_RIGID/LConn2 -- bracesb1_2_RIGID/LConn1
  bracesb1_1_RIGID/LConn1 -- bracesb1_7_RIGID/LConn5
  bracesb2_1_RIGID/LConn2 -- bracesb2_2_RIGID/LConn1
  bracesb2_1_RIGID/LConn1 -- link4l_1_RIGID/LConn3
  bracesb3_1_RIGID/LConn2 -- bracesb3_2_RIGID/LConn1
  bracesb3_1_RIGID/LConn3 -- link3l_1_RIGID/LConn1
  bracesb3_1_RIGID/LConn1 -- bulkheads3_2_RIGID/LConn2
  bracesb6_8_RIGID/LConn1 -- rear_torso_l_1_RIGID/LConn4
  bracesb5_1_RIGID/LConn3 -- bracesb5_2_RIGID/LConn1
  Bracket_6_RIGID/LConn1 -- Spacer_1_RIGID3/LConn2 -- link5l_1_RIGID/LConn3 -- Spring_Pin_1_8_in_OD_1_4_in_L_22_RIGID/LConn1 -- Spring_Pin_1_8_in_OD_1_4_in_L_18_RIGID2/LConn1 -- Spacer_1_RIGID24/LConn1 -- Set_Screw_4_1_4_in_18_RIGID/LConn1 -- Set_Screw_4_1_4_in_10_RIGID/LConn1 -- Screw_8_3_4_in_1_RIGID4/LConn1 -- Screw_8_3_4_in_1_RIGID2/LConn1 -- Screw_8_1_2_in_1_RIGID8/LConn1 -- Screw_8_1_2_in_1_RIGID17/LConn1 -- Lock_tabs_1_RIGID5/LConn1 -- Lock_tabs_1_RIGID2/LConn1 -- Hinge_6_RIGID/LConn1 -- Bracket_19_RIGID/LConn1 -- Hinge_1_RIGID2/LConn1 -- Spring_Pin_1_8_in_OD_1_4_in_L_5_RIGID/LConn1 -- Spring_Pin_1_8_in_OD_1_4_in_L_5_RIGID2/LConn1 -- Spring_Pin_1_8_in_OD_1_4_in_L_5_RIGID3/LConn1 -- Spring_Pin_1_8_in_OD_1_4_in_L_8_RIGID1/LConn1 -- Spring_Pin_3_32_in_OD_3_16_in_L_1_RIGID10/LConn1 -- Spring_Pin_3_32_in_OD_3_16_in_L_1_RIGID11/LConn1 -- Spring_Pin_3_32_in_OD_3_16_in_L_1_RIGID2/LConn1 -- Spring_Pin_3_32_in_OD_3_16_in_L_1_RIGID3/LConn1 -- Spring_Pin_3_32_in_OD_3_16_in_L_1_RIGID5/LConn1 -- Spring_Pin_3_32_in_OD_3_16_in_L_1_RIGID8/LConn1 -- Standoff_1_RIGID/LConn1 -- Washer_8_1_RIGID2/LConn1 -- Washer_8_1_RIGID22/LConn1 -- Washer_8_1_RIGID23/LConn1 -- Washer_8_1_RIGID5/LConn1 -- link5r_1_RIGID/LConn1
  bracesb6_4_RIGID/LConn1 -- bracesb6_5_RIGID/LConn1
  bracesb2_3_RIGID/LConn1 -- link4r_1_RIGID/LConn1
  bracesb7_3_RIGID/LConn2 -- bracesb7_4_RIGID/LConn1
  bracesb4_3_RIGID/LConn1 -- link2r_1_RIGID/LConn1
  bracesb1_5_RIGID/LConn1 -- bracesb1_7_RIGID/LConn4
  bracesb7_5_RIGID/LConn1 -- bracesb7_6_RIGID/LConn1
  bracesb4_1_RIGID/LConn2 -- bracesb4_2_RIGID/LConn1
  bracesb4_1_RIGID/LConn1 -- link2l_1_RIGID/LConn2
  Cylindrical3/LConn1 -- Frame_Part_2_RIGID1/RConn2
  Cylindrical3/RConn1 -- Spacer_1_RIGID21/LConn1
  link4l_1_RIGID/LConn1 -- link4r_1_RIGID/LConn2
  Revolute3/LConn1 -- Spacer_1_RIGID25/RConn1
  Revolute3/RConn1 -- link3l_1_RIGID/LConn5
  Revolute11/LConn1 -- link2l_1_RIGID/RConn1
  Lock_tabs_1_RIGID10/LConn2 -- Revolute11/RConn1
  Revolute2/LConn1 -- link2l_1_RIGID/RConn2
  Revolute2/RConn1 -- Spacer_1_RIGID4/LConn1
  Revolute1/LConn1 -- link1l_1_RIGID/RConn1
  Revolute1/RConn1 -- Spacer_1_RIGID9/LConn1
  Cylindrical4/LConn1 -- Frame_Part_2_RIGID1/RConn1
  Cylindrical4/RConn1 -- Lock_tabs_1_RIGID3/LConn2
  Bracket_14_RIGID/LConn1 -- Lock_tabs_1_RIGID8/LConn2 -- Spacer_1_RIGID14/LConn2 -- Bracket_1_RIGID/LConn1 -- Bracket_18_RIGID/LConn1 -- Bracket_17_RIGID/LConn1 -- Bracket_15_RIGID/LConn1 -- Bracket_11_RIGID/LConn1 -- Lock_tabs_1_RIGID10/LConn1 -- Lock_tabs_1_RIGID3/LConn1 -- Hinge_1_RIGID/LConn1 -- Bracket_22_RIGID/LConn1 -- Bracket_4_RIGID/LConn1 -- Frame_Part_1_RIGID1/LConn1 -- Frame_Part_2_RIGID/LConn1 -- Hinge_11_RIGID/LConn1 -- Hinge_1_RIGID1/LConn1 -- Hinge_4_RIGID/LConn1 -- Hinge_9_RIGID/LConn1 -- Lock_tabs_1_RIGID11/LConn1 -- Lock_tabs_1_RIGID4/LConn1 -- Lock_tabs_1_RIGID6/LConn1 -- Lock_tabs_1_RIGID7/LConn1 -- Lock_tabs_1_RIGID9/LConn1 -- Screw_8_1_2_in_1_RIGID10/LConn1 -- Screw_8_1_2_in_1_RIGID11/LConn1 -- Screw_8_1_2_in_1_RIGID15/LConn1 -- Screw_8_1_2_in_1_RIGID16/LConn1 -- Screw_8_1_2_in_1_RIGID2/LConn1 -- Screw_8_1_2_in_1_RIGID6/LConn1 -- Screw_8_1_2_in_1_RIGID7/LConn1 -- Screw_8_1_2_in_1_RIGID9/LConn1 -- Screw_8_3_4_in_1_RIGID/LConn1 -- Screw_8_3_4_in_1_RIGID5/LConn1 -- Set_Screw_4_1_4_in_12_RIGID/LConn1 -- Set_Screw_4_1_4_in_14_RIGID/LConn1 -- Set_Screw_4_1_4_in_16_RIGID/LConn1 -- Set_Screw_4_1_4_in_19_RIGID/LConn1 -- Set_Screw_4_1_4_in_21_RIGID/LConn1 -- Set_Screw_4_1_4_in_22_RIGID/LConn1 -- Set_Screw_4_1_4_in_23_RIGID/LConn1 -- Set_Screw_4_1_4_in_3_RIGID/LConn1 -- Spacer_1_RIGID/LConn1 -- Spacer_1_RIGID15/LConn1 -- Spacer_1_RIGID16/LConn1 -- Spacer_1_RIGID17/LConn1 -- Spacer_1_RIGID19/LConn1 -- Spacer_1_RIGID20/LConn1 -- Spacer_1_RIGID8/LConn1 -- Spring_Pin_1_8_in_OD_1_4_in_L_10_RIGID/LConn1 -- Spring_Pin_1_8_in_OD_1_4_in_L_10_RIGID1/LConn1 -- Spring_Pin_1_8_in_OD_1_4_in_L_13_RIGID2/LConn1 -- Spring_Pin_1_8_in_OD_1_4_in_L_14_RIGID/LConn1 -- Spring_Pin_1_8_in_OD_1_4_in_L_14_RIGID1/LConn1 -- Spring_Pin_1_8_in_OD_1_4_in_L_15_RIGID/LConn1 -- Spring_Pin_1_8_in_OD_1_4_in_L_15_RIGID2/LConn1 -- Spring_Pin_1_8_in_OD_1_4_in_L_16_RIGID1/LConn1 -- Spring_Pin_1_8_in_OD_1_4_in_L_17_RIGID2/LConn1 -- Spring_Pin_1_8_in_OD_1_4_in_L_18_RIGID/LConn1 -- Spring_Pin_1_8_in_OD_1_4_in_L_19_RIGID1/LConn1 -- Spring_Pin_1_8_in_OD_1_4_in_L_19_RIGID2/LConn1 -- Spring_Pin_1_8_in_OD_1_4_in_L_1_RIGID2/LConn1 -- Spring_Pin_1_8_in_OD_1_4_in_L_20_RIGID/LConn1 -- Spring_Pin_1_8_in_OD_1_4_in_L_20_RIGID1/LConn1 -- Spring_Pin_1_8_in_OD_1_4_in_L_20_RIGID2/LConn1 -- Spring_Pin_1_8_in_OD_1_4_in_L_2_RIGID2/LConn1 -- Spring_Pin_1_8_in_OD_1_4_in_L_3_RIGID/LConn1 -- Spring_Pin_1_8_in_OD_1_4_in_L_4_RIGID/LConn1 -- Spring_Pin_1_8_in_OD_1_4_in_L_4_RIGID3/LConn1 -- Spring_Pin_1_8_in_OD_1_4_in_L_6_RIGID3/LConn1 -- Spring_Pin_1_8_in_OD_1_4_in_L_7_RIGID/LConn1 -- Spring_Pin_1_8_in_OD_1_4_in_L_9_RIGID/LConn1 -- Spring_Pin_1_8_in_OD_1_4_in_L_9_RIGID2/LConn1 -- Spring_Pin_3_32_in_OD_3_16_in_L_1_RIGID/LConn1 -- Spring_Pin_3_32_in_OD_3_16_in_L_1_RIGID1/LConn1 -- Spring_Pin_3_32_in_OD_3_16_in_L_1_RIGID4/LConn1 -- Spring_Pin_3_32_in_OD_3_16_in_L_1_RIGID6/LConn1 -- Spring_Pin_3_32_in_OD_3_16_in_L_1_RIGID7/LConn1 -- Spring_Pin_3_32_in_OD_3_16_in_L_1_RIGID9/LConn1 -- Washer_8_1_RIGID/LConn1 -- Washer_8_1_RIGID1/LConn1 -- Washer_8_1_RIGID12/LConn1 -- Washer_8_1_RIGID13/LConn1 -- Washer_8_1_RIGID14/LConn1 -- Washer_8_1_RIGID15/LConn1 -- Washer_8_1_RIGID16/LConn1 -- Washer_8_1_RIGID24/LConn1 -- Washer_8_1_RIGID3/LConn1 -- Washer_8_1_RIGID6/LConn1
  bracesb6_1_RIGID/LConn4 -- rear_torso_l_1_RIGID/LConn1
  bracesb7_7_RIGID/LConn1 -- rear_torso_l_1_RIGID/LConn3
  Revolute7/LConn1 -- rear_torso_l_1_RIGID/RConn1
  Revolute7/RConn1 -- Spacer_1_RIGID13/LConn1
  bracesb1_3_RIGID/LConn1 -- bracesb1_4_RIGID/LConn1
  bracesb5_1_RIGID/LConn2 -- bracesb5_3_RIGID/LConn1
  bracesb1_3_RIGID/LConn2 -- bracesb1_7_RIGID/LConn3
  bracesb1_7_RIGID/LConn6 -- link5l_1_RIGID/LConn1
  bracesb1_7_RIGID/LConn1 -- bulkheads2_2_RIGID/LConn2
  bracesb1_6_RIGID/LConn1 -- bracesb1_7_RIGID/LConn2
  bulkheads4_2_RIGID/LConn1 -- bulkheads4_1_RIGID/LConn1 -- bulkheads4_3_RIGID/LConn1 -- bulkheads4_4_RIGID/LConn1 -- bulkheads4_5_RIGID/LConn1
  Revolute4/LConn1 -- link4l_1_RIGID/RConn1
  Revolute4/RConn1 -- Spacer_1_RIGID14/LConn1
  bracesb6_1_RIGID/LConn2 -- bracesb6_4_RIGID/LConn2
  bracesb6_1_RIGID/LConn1 -- bracesb6_6_RIGID/LConn2
  bracesb6_6_RIGID/LConn1 -- bracesb6_7_RIGID/LConn1
  Cylindrical5/LConn1 -- link5l_1_RIGID/RConn1
  Cylindrical5/RConn1 -- Lock_tabs_1_RIGID8/LConn1
  bracesb5_1_RIGID/LConn1 -- bulkheads4_2_RIGID/LConn2
  bracesb5_1_RIGID/LConn4 -- link1l_1_RIGID/LConn1
  Revolute6/LConn1 -- Spacer_1_RIGID12/RConn1
  Bracket_13_RIGID/LConn1 -- Spacer_1_RIGID21/LConn2 -- Spacer_1_RIGID4/LConn2 -- Spacer_1_RIGID13/LConn2 -- Spacer_1_RIGID22/LConn1 -- Spacer_1_RIGID10/LConn1 -- Set_Screw_4_1_4_in_7_RIGID/LConn1 -- Set_Screw_4_1_4_in_6_RIGID/LConn1 -- Set_Screw_4_1_4_in_2_RIGID/LConn1 -- Set_Screw_4_1_4_in_24_RIGID/LConn1 -- Set_Screw_4_1_4_in_13_RIGID/LConn1 -- Set_Screw_4_1_4_in_11_RIGID/LConn1 -- Screw_8_3_4_in_1_RIGID3/LConn1 -- Screw_8_3_4_in_1_RIGID1/LConn1 -- Screw_8_1_2_in_1_RIGID5/LConn1 -- Screw_8_1_2_in_1_RIGID18/LConn1 -- Screw_8_1_2_in_1_RIGID13/LConn1 -- Screw_8_1_2_in_1_RIGID12/LConn1 -- Lock_tabs_1_RIGID13/LConn1 -- Lock_tabs_1_RIGID12/LConn1 -- Lock_tabs_1_RIGID1/LConn1 -- Lock_tabs_1_RIGID/LConn1 -- Hinge_8_RIGID/LConn1 -- Hinge_13_RIGID/LConn1 -- Hinge_10_RIGID/LConn1 -- Frame_Part_2_RIGID2/LConn1 -- Frame_Part_1_RIGID2/LConn1 -- Bracket_8_RIGID/LConn1 -- Bracket_21_RIGID/LConn1 -- Bracket_20_RIGID/LConn1 -- Bracket_16_RIGID/LConn1 -- Bracket_10_RIGID/LConn1 -- Spacer_1_RIGID5/LConn1 -- Spring_Pin_1_8_in_OD_1_4_in_L_10_RIGID2/LConn1 -- Spring_Pin_1_8_in_OD_1_4_in_L_10_RIGID3/LConn1 -- Spring_Pin_1_8_in_OD_1_4_in_L_11_RIGID2/LConn1 -- Spring_Pin_1_8_in_OD_1_4_in_L_12_RIGID/LConn1 -- Spring_Pin_1_8_in_OD_1_4_in_L_12_RIGID3/LConn1 -- Spring_Pin_1_8_in_OD_1_4_in_L_13_RIGID/LConn1 -- Spring_Pin_1_8_in_OD_1_4_in_L_14_RIGID2/LConn1 -- Spring_Pin_1_8_in_OD_1_4_in_L_15_RIGID1/LConn1 -- Spring_Pin_1_8_in_OD_1_4_in_L_16_RIGID/LConn1 -- Spring_Pin_1_8_in_OD_1_4_in_L_21_RIGID/LConn1 -- Spring_Pin_1_8_in_OD_1_4_in_L_2_RIGID/LConn1 -- Spring_Pin_1_8_in_OD_1_4_in_L_3_RIGID3/LConn1 -- Spring_Pin_1_8_in_OD_1_4_in_L_5_RIGID1/LConn1 -- Spring_Pin_1_8_in_OD_1_4_in_L_6_RIGID1/LConn1 -- Spring_Pin_1_8_in_OD_1_4_in_L_6_RIGID2/LConn1 -- Spring_Pin_1_8_in_OD_1_4_in_L_7_RIGID3/LConn1 -- Spring_Pin_1_8_in_OD_1_4_in_L_8_RIGID/LConn1 -- Spring_Pin_1_8_in_OD_1_4_in_L_9_RIGID1/LConn1 -- Washer_8_1_RIGID10/LConn1 -- Washer_8_1_RIGID18/LConn1 -- Washer_8_1_RIGID19/LConn1 -- Washer_8_1_RIGID21/LConn1 -- Washer_8_1_RIGID25/LConn1 -- Washer_8_1_RIGID8/LConn1
  Revolute6/RConn1 -- link1l_1_RIGID/LConn3
  Hinge_1_RIGID2/LConn2 -- F/RConn1
  link3l_1_RIGID/LConn3 -- F1/RConn1
  Spacer_1_RIGID3/LConn1 -- F2/RConn1
  Hinge_3_RIGID/LConn2 -- F3/RConn1
  Hinge_1_RIGID/LConn2 -- F4/RConn1
  link1l_1_RIGID/LConn4 -- F5/RConn1
  Spacer_1_RIGID12/LConn2 -- F6/RConn1
  link5l_1_RIGID/LConn2 -- F7/RConn1
  link4l_1_RIGID/LConn2 -- F8/RConn1
  bulkheads2_2_RIGID/LConn1 -- bulkheads2_1_RIGID/LConn1 -- bulkheads2_3_RIGID/LConn1 -- bulkheads2_5_RIGID/LConn1 -- bulkheads2_4_RIGID/LConn1
  Transform/RConn1 -- rear_torso_l_1_RIGID/LConn2
  ReferenceFrame/RConn1 -- Transform/LConn1
  link2l_1_RIGID/LConn1 -- link2r_1_RIGID/LConn2
  S4/RConn1 -- Spacer_1_RIGID18/RConn1
